simulink model "Farm_FaultBottomBar"  (R2019a)
settings: Solver=ode1  StartTime=0.0  StopTime=1.5  FixedStep=Ts_Power  RelTol=1e-3
PostLoadFcn:
  | %% Init for wind PnO models - global system parameters
  | OVERRIDE_SSN_MEMORY_LIMIT=1;
  | Ts=50e-6;
  | % Ts=50e-10;
  | Ts_Power=Ts;
  | Ts_Control=2*Ts;
  | freq = 50;
  | Fnom=freq;
  | Vac=400e3;
InitFcn:
  | %% Init for wind PnO models - global system parameters
  | OVERRIDE_SSN_MEMORY_LIMIT=1;
  | Ts=50e-6;
  | % Ts=50e-10;
  | Ts_Power=Ts;
  | Ts_Control=2*Ts;
  | freq = 50;
  | Fnom=freq;
  | Vac=400e3;
undefined symbols (not defined in the file or in its folder): D11, Delta, den, DiscIntNeverNeededParam, dx, find_system, gcbh, num, out_Buses, out_WindFarms, sps_rtmsupport
libraries: powerlib x283, simulink x112, powerlib_meascontrol x112, eeSinusoidalMeasurement x76, spsVIMeasurementModel x66, elements x52, simulink_extras x44, eePowerMeasurement x27
(part 17 of 28)

== system Farm_FaultBottomBar/SM_WT1/Wind Type IV Detailed v2.1 - 2/Control/Measurement and Transformation ==
  note: Inputs / filtering
  note: P,Q & V
  note: PLL
  note: Outputs
  note: Check for normal voltage
  note: Protection against unstable grid events
  note: Check for normal frequency
  note: Block forever in case of
      | persistent system overvoltage
  Vabc_grid : Inport
  Iabc_gc : Inport  Port=2
  IL : Inport  Port=3
  Vdc : Inport  Port=4
  Qref : Inport  Port=5
  C_var_filter : Gain  Gain=C_var_filter  SaturateOnIntegerOverflow=on  OutDataTypeStr=Inherit: Same as input  ParamDataTypeStr=Inherit: Same as input
  C_var_filter/Q : Gain  Gain=C_var_filter/Q_filter  SaturateOnIntegerOverflow=on  OutDataTypeStr=Inherit: Same as input  ParamDataTypeStr=Inherit: Same as input
  Compare To Constant1 : simulink/Logic and Bit Operations/Compare To Constant  relop=<  const=0.5  OutDataTypeStr=boolean
  Compare To Constant3 : simulink/Logic and Bit Operations/Compare To Constant  relop=<  const=0.5  OutDataTypeStr=boolean
  Constant : Constant  Value=Vnom
  Constant1 : Constant  Value=Vnom/sqrt(3)*sqrt(2)
  Constant2 : Constant  Value=20
  Constant3 : Constant  SampleTime=Ts
  Constant4 : Constant  SampleTime=Ts
  Digital Clock1 : DigitalClock  SampleTime=Ts
  Digital Clock2 : DigitalClock  SampleTime=Ts
  Discrete 3-phase PLL-Driven Positive-Sequence Active & Reactive Power : Subsystem  mask(Discrete 3-phase PLL-Driven Positive-Sequence Active & Reactive Power){Finit=freq, Fmin=freq*45/60, Par_Vinit=[Vnom/sqrt(3)*sqrt(2) 30], Par_Iinit=[Pnom/sqrt(3)/Vnom*sqrt(2) -10], Ts=Ts}
      mask prompts: Finit "Initial frequency (Hz):"; Fmin "Minimum frequency (Hz):"; Par_Vinit "Voltage initial input: [ Mag  Phase(Degrees) ]"; Par_Iinit "Current initial input: [ Mag  Phase(Degrees) ]"; Ts "Sample time:"
      mask help:
      | This discrete block measures the 3-phase active power P and reactive power Q  associated with a periodic set of 3-phase voltages and currents which may contain harmonics. P and Q are calculated by evaluating the fundamental values (positive-sequence) of the input voltages and currents with a running window over one cycle of the specified frequency (port Freq).
      |  Input port "Sin_Cos" (a two-dimension signal) provides the reference frame required for the computation.
      |
      | input 1: must give the frequency of the fundamental (Hz)
      | Input 2: must contain a  [sin(wt)  cos(wt)] two dimension signal , where w is the rotation speed (rad/s) of the reference frame used for the computation..
      | input 3: Vectorized 3-phase  instantaneous voltage (Vabc)
      | input 4: Vectorized 3-phase instantaneous current (Iabc)
      |
      | Output 1: Vector [Mag_V Mag_I] of the fundamental values (Magnitude) of the voltage & current (peak values of the positive-sequence)
      | Output 2: 3-phase PQ measurement vector [P(W) Q (var)] evaluated at the specified frequency. Current flowing into an RL circuit will produce  positive active and reactive powers.
      |
      | For the first cycle of simulation, the outputs are held constant using the values specified by the parameters "Initial input".
      | he value of the parameter "Minimum frequency" is used to determine the buffer size of the "Variable Transport Delay" block found inside this subsystem.
      mask init:
      | power_initmask();
      settings: OpenFcn=power_openblockproxy();
  Divide : Product  Inputs=*/
  Filter : Subsystem  mask{Freq=Freq_filter, Zeta=Zeta_filter, Ts=Ts}
      mask prompts: Freq "Cut-off frequency (Hz):"; Zeta "Damping factor Zeta:"; Ts "Sample time"
  Gain : Gain  Gain=1.4
  Less Than : RelationalOperator  Operator=>  OutDataTypeStr=boolean  RndMeth=Simplest
  Less Than1 : RelationalOperator  Operator=>  OutDataTypeStr=boolean  RndMeth=Simplest
  Logical Operator : Logic  AllPortsSameDT=off  OutDataTypeStr=boolean
  Math Function1 : Math  Operator=square  SaturateOnIntegerOverflow=on
  Max : MinMax  Inputs=2
  Memory : Memory  InitialCondition=1
  Second-Order Filter1 : powerlib_meascontrol/Filters/Second-Order Filter  FilterType=Lowpass  Fo=50  Zeta=0.707  Ts=Ts  Initialize=off  Vac_Init="[0,  0,  60]"  Vdc_Init=0  PlotResponse=off  FreqRange=[0, 500, 1]
      settings: SourceProductBaseCode=PS
  Selector1 : Selector  InputPortWidth=2  IndexOptions=Index vector (dialog)  Indices=1  OutputSizes=1
  Selector2 : Selector  InputPortWidth=2  IndexOptions=Index vector (dialog)  Indices=1  OutputSizes=1
  Selector3 : Selector  InputPortWidth=2  IndexOptions=Index vector (dialog)  Indices=2  OutputSizes=1
  "Sinusoidal Measurement (PLL, Three-Phase)" : eeSinusoidalMeasurement/Sinusoidal Measurement (PLL, Three-Phase)  Kp_LF=200*0.1  Ki_LF=2000*0.1  F0=freq  Theta0=0  Ts=-1
      settings: SourceProductBaseCode=PS
  Sum : Sum  Inputs=|-+
  Sum1 : Sum  Inputs=|++
  Switch1 : Switch  Criteria=u2 > Threshold
  Switch2 : Switch  Criteria=u2 > Threshold
  Terminator : Terminator
  V->pu : Gain  Gain=1/(Vnom/sqrt(3)*sqrt(2))  SaturateOnIntegerOverflow=on  OutDataTypeStr=Inherit: Same as input  ParamDataTypeStr=Inherit: Same as input
  W->pu : Gain  Gain=-1/Pnom  SaturateOnIntegerOverflow=on  OutDataTypeStr=Inherit: Same as input  ParamDataTypeStr=Inherit: Same as input
  pu->A : Gain  Gain=Pnom/sqrt(3)/Vnom*sqrt(2)  SaturateOnIntegerOverflow=on  OutDataTypeStr=Inherit: Same as input  ParamDataTypeStr=Inherit: Same as input
  pu->V : Gain  Gain=Vnom/sqrt(3)*sqrt(2)  SaturateOnIntegerOverflow=on  OutDataTypeStr=Inherit: Same as input  ParamDataTypeStr=Inherit: Same as input
  "var->pu " : Gain  Gain=-1/Pnom  SaturateOnIntegerOverflow=on  OutDataTypeStr=Inherit: Same as input  ParamDataTypeStr=Inherit: Same as input
  "IL " : Outport  VectorParamsAs1DForOutWhenUnconnected=on
  Theta_PLL : Outport  Port=2  VectorParamsAs1DForOutWhenUnconnected=on
  Pmeas : Outport  Port=3  VectorParamsAs1DForOutWhenUnconnected=on
  Qmeas : Outport  Port=4  VectorParamsAs1DForOutWhenUnconnected=on
  Vmag : Outport  Port=5  VectorParamsAs1DForOutWhenUnconnected=on
  Vdc_meas : Outport  Port=6  VectorParamsAs1DForOutWhenUnconnected=on
  Qref_pu : Outport  Port=7  VectorParamsAs1DForOutWhenUnconnected=on
  Vnormal : Outport  Port=8  VectorParamsAs1DForOutWhenUnconnected=on
  wires:
  [IL] -> "IL "/1
  Filter/3("IL ") -> [IL]
  IL/1 -> Filter/3(IL)
  Sum1/1 -> W->pu/1
  C_var_filter/Q/1 -> Sum1/2
  Selector1/1 -> Sum1/1
  Math Function1/1 -> C_var_filter/1, C_var_filter/Q/1
  Sum/1 -> "var->pu "/1  "Q meas"
  C_var_filter/1 -> Sum/1
  Selector3/1 -> Sum/2  "Q grid"
  Divide/1 -> Math Function1/1
  Constant1/1 -> Divide/2
  [V_volt] -> Divide/1
  Iabc_gc/1 -> Filter/2(Iabc_grid_conv)
  Filter/5("Qref ") -> [Qref]
  Filter/4("Vdc ") -> [Vdc_meas]
  Filter/2("Iabc_grid_conv ") -> [Iabc_gc]
  Filter/1("Vabc_grid ") -> [Vabc_grid]
  Qref/1 -> Filter/5(Qref)
  Vdc/1 -> Filter/4(Vdc)
  Vabc_grid/1 -> Filter/1(Vabc_grid)
  Discrete 3-phase PLL-Driven Positive-Sequence Active & Reactive Power/2(P_Q) -> [PQ]
  [Iabc_gc] -> pu->A/1
  [Qref] -> Qref_pu/1
  [Vdc_meas] -> Vdc_meas/1
  [PQ] -> Selector1/1
  pu->A/1 -> Discrete 3-phase PLL-Driven Positive-Sequence Active & Reactive Power/4(Iabc)
  [Vmeas] -> Vmag/1
  [Pmeas] -> Pmeas/1
  [Theta] -> Theta_PLL/1
  [Vabc_grid] -> "Sinusoidal Measurement (PLL, Three-Phase)"/1
  [Theta] -> Discrete 3-phase PLL-Driven Positive-Sequence Active & Reactive Power/2(w)
  "Sinusoidal Measurement (PLL, Three-Phase)"/2 -> [Theta]
  W->pu/1 -> [Pmeas]
  pu->V/1 -> Discrete 3-phase PLL-Driven Positive-Sequence Active & Reactive Power/3(Vabc)
  "Sinusoidal Measurement (PLL, Three-Phase)"/1 -> [Freq]
  Discrete 3-phase PLL-Driven Positive-Sequence Active & Reactive Power/1(Mag_V_I) -> Selector2/1
  [V_volt] -> V->pu/1
  V->pu/1 -> [Vmeas]
  [PQ] -> Selector3/1
  "var->pu "/1 -> [Qmeas]  "Q meas pu"
  [Qmeas] -> Qmeas/1
  "Sinusoidal Measurement (PLL, Three-Phase)"/3 -> Terminator/1
  Selector2/1 -> [V_volt]  "V volt"
  [Vabc_grid] -> pu->V/1
  [Vnormal] -> Vnormal/1
  [Freq] -> Discrete 3-phase PLL-Driven Positive-Sequence Active & Reactive Power/1(Freq)
  [V_volt] -> Second-Order Filter1/1
  Constant2/1 -> Less Than1/2  "20 Hz"
  [Freq] -> Less Than1/1  "Freq"
  Memory/1 -> Max/2
  Gain/1 -> Less Than/1
  Second-Order Filter1/1 -> Less Than/2
  Constant/1 -> Gain/1
  Max/1 -> [Vnormal], Memory/1
  Logical Operator/1 -> Max/1
  Constant3/1 -> Switch2/1
  Digital Clock1/1 -> Compare To Constant3/1
  Compare To Constant3/1 -> Switch2/2
  Less Than/1 -> Switch2/3
  Switch2/1 -> Logical Operator/1  "test1"
  Digital Clock2/1 -> Compare To Constant1/1
  Constant4/1 -> Switch1/1
  Less Than1/1 -> Switch1/3  "Comparator freq"
  Switch1/1 -> Logical Operator/2  "test2"
  Compare To Constant1/1 -> Switch1/2

== system Farm_FaultBottomBar/SM_WT1/Wind Type IV Detailed v2.1 - 2/Control/PI_P ==
  u : Inport
  Enable : EnablePort
  Discrete PID Controller2 : simulink/Continuous/PID Controller  Controller=PI  Form=Parallel  TimeDomain=Discrete-time  SampleTime=-1  IntegratorMethod=Forward Euler  FilterMethod=Forward Euler  ControllerParametersSource=internal  P=5  I=30  D=2  UseFilter=on  N=100  TunerSelectOption=Transfer Function Based (PID Tuner App)  InitialConditionSource=internal  InitialConditionForIntegrator=0  InitialConditionForFilter=0  DifferentiatorICPrevScaledInput=0  ExternalReset=none  TrackingMode=off  Kt=1  LimitOutput=on  UpperSaturationLimit=0.8  LowerSaturationLimit=-0.8  LinearizeAsGain=off  AntiWindupMode=none  Kb=1  POutMin=[]  POutMax=[]  IOutMin=[]  IOutMax=[]  DOutMin=[]  DOutMax=[]  NOutMin=[]  NOutMax=[]  SumOutMin=[]  SumOutMax=[]  SaturationOutMin=[]  SaturationOutMax=[]  PParamMin=[]  PParamMax=[]  IParamMin=[]  IParamMax=[]  DParamMin=[]  DParamMax=[]  NParamMin=[]  NParamMax=[]  KbParamMin=[]  KbParamMax=[]  KtParamMin=[]  KtParamMax=[]  KbOutMin=[]  KbOutMax=[]  KtOutMin=[]  KtOutMax=[]  IntegratorOutMin=[]  IntegratorOutMax=[]  FilterOutMin=[]  FilterOutMax=[]  SumI1OutMin=[]  SumI1OutMax=[]  SumI2OutMin=[]  SumI2OutMax=[]  SumI3OutMin=[]  SumI3OutMax=[]  SumI4OutMin=[]  SumI4OutMax=[]  SumDOutMin=[]  SumDOutMax=[]  DifferentiatorOutMin=[]  DifferentiatorOutMax=[]  FilterDiffOutCoefMin=[]  FilterDiffOutCoefMax=[]  ReciprocalOutMin=[]  ReciprocalOutMax=[]  SumDenOutMin=[]  SumDenOutMax=[]  SumNumOutMin=[]  SumNumOutMax=[]  DivideOutMin=[]  DivideOutMax=[]  IntegratorContinuousStateAttributes=''  IntegratorStateMustResolveToSignalObject=off  IntegratorRTWStateStorageClass=Auto  FilterContinuousStateAttributes=''  FilterStateMustResolveToSignalObject=off  FilterRTWStateStorageClass=Auto  ParallelPVariant=InternalParameters  IdealPVariant=Disabled  IVariant=InternalParameters  DVariant=Disabled  IntegratorVariant=Discrete  SatVariant=Enabled  AWVariant=Passthrough  PCopyVariant=Disabled  TRVariant=Disabled  FdbkBlocksVariant=Forward  IdealPFdbkVariant=Disabled  SatFdbkVariant=Disabled  DerivativeFilterVariant=Disabled  NVariant=Disabled  NCopyVariant=Disabled_SignalSpec  FilterICVariant=Disabled  IntegratorICVariant=InternalICs  ExternalResetVariant=Disabled  TRSumVariant=Passthrough  SumFdbkVariant=Disabled  SumVariant=Sum_PI
  PI_out : Outport  VectorParamsAs1DForOutWhenUnconnected=on
  wires:
  Discrete PID Controller2/1 -> PI_out/1  "d PI_out"
  u/1 -> Discrete PID Controller2/1

== system Farm_FaultBottomBar/SM_WT1/Wind Type IV Detailed v2.1 - 2/Control/PI_Q ==
  Qerr : Inport
  Enable : EnablePort
  Discrete PID Controller1 : simulink/Continuous/PID Controller  Controller=PI  Form=Parallel  TimeDomain=Discrete-time  SampleTime=-1  IntegratorMethod=Forward Euler  FilterMethod=Forward Euler  ControllerParametersSource=internal  P=0.5  I=8  D=2  UseFilter=on  N=100  TunerSelectOption=Transfer Function Based (PID Tuner App)  InitialConditionSource=internal  InitialConditionForIntegrator=0  InitialConditionForFilter=0  DifferentiatorICPrevScaledInput=0  ExternalReset=none  TrackingMode=off  Kt=1  LimitOutput=off  UpperSaturationLimit=inf  LowerSaturationLimit=-inf  LinearizeAsGain=off  AntiWindupMode=none  Kb=1  POutMin=[]  POutMax=[]  IOutMin=[]  IOutMax=[]  DOutMin=[]  DOutMax=[]  NOutMin=[]  NOutMax=[]  SumOutMin=[]  SumOutMax=[]  SaturationOutMin=[]  SaturationOutMax=[]  PParamMin=[]  PParamMax=[]  IParamMin=[]  IParamMax=[]  DParamMin=[]  DParamMax=[]  NParamMin=[]  NParamMax=[]  KbParamMin=[]  KbParamMax=[]  KtParamMin=[]  KtParamMax=[]  KbOutMin=[]  KbOutMax=[]  KtOutMin=[]  KtOutMax=[]  IntegratorOutMin=[]  IntegratorOutMax=[]  FilterOutMin=[]  FilterOutMax=[]  SumI1OutMin=[]  SumI1OutMax=[]  SumI2OutMin=[]  SumI2OutMax=[]  SumI3OutMin=[]  SumI3OutMax=[]  SumI4OutMin=[]  SumI4OutMax=[]  SumDOutMin=[]  SumDOutMax=[]  DifferentiatorOutMin=[]  DifferentiatorOutMax=[]  FilterDiffOutCoefMin=[]  FilterDiffOutCoefMax=[]  ReciprocalOutMin=[]  ReciprocalOutMax=[]  SumDenOutMin=[]  SumDenOutMax=[]  SumNumOutMin=[]  SumNumOutMax=[]  DivideOutMin=[]  DivideOutMax=[]  IntegratorContinuousStateAttributes=''  IntegratorStateMustResolveToSignalObject=off  IntegratorRTWStateStorageClass=Auto  FilterContinuousStateAttributes=''  FilterStateMustResolveToSignalObject=off  FilterRTWStateStorageClass=Auto  ParallelPVariant=InternalParameters  IdealPVariant=Disabled  IVariant=InternalParameters  DVariant=Disabled  IntegratorVariant=Discrete  SatVariant=Disabled  AWVariant=Passthrough  PCopyVariant=Disabled  TRVariant=Disabled  FdbkBlocksVariant=Forward  IdealPFdbkVariant=Disabled  SatFdbkVariant=Disabled  DerivativeFilterVariant=Disabled  NVariant=Disabled  NCopyVariant=Disabled_SignalSpec  FilterICVariant=Disabled  IntegratorICVariant=InternalICs  ExternalResetVariant=Disabled  TRSumVariant=Passthrough  SumFdbkVariant=Disabled  SumVariant=Sum_PI
  PI_out : Outport  VectorParamsAs1DForOutWhenUnconnected=on
  wires:
  Discrete PID Controller1/1 -> PI_out/1  "q PI_out"
  Qerr/1 -> Discrete PID Controller1/1

== system Farm_FaultBottomBar/SM_WT1/Wind Type IV Detailed v2.1 - 2/Control/Pulse Generator1 ==
  Duty_Cycle : Inport
  Add : Sum  Inputs=-+
  Constant3 : Constant
  Constant4 : Constant  Value=0
  Digital Clock : DigitalClock  SampleTime=Ts
  Divide2 : Product  Inputs=**
  Divide3 : Product  Inputs=**
  Math Function : Math  Operator=mod  SaturateOnIntegerOverflow=on
  Nb_of_samples_by_cycle : Constant  Value=1/Freq_sawtooth/Ts
  Relational Operator1 : RelationalOperator  Operator=>  OutDataTypeStr=boolean  RndMeth=Nearest
  Rounding Function1 : Rounding  Operator=round
  Switch : Switch  Threshold=0.5
  Ts : Constant  Value=Ts
  Pulse : Outport  VectorParamsAs1DForOutWhenUnconnected=on
  wires:
  Switch/1 -> Pulse/1
  Add/1 -> Divide2/2
  Digital Clock/1 -> Math Function/1
  Ts/1 -> Add/1, Divide3/1
  Rounding Function1/1 -> Divide3/2  "Nb_of_samples_by_cycle"
  Duty_Cycle/1 -> Divide2/1
  Divide3/1 -> Math Function/2, Add/2  "Period_of_cycle"
  Divide2/1 -> Relational Operator1/1
  Nb_of_samples_by_cycle/1 -> Rounding Function1/1
  Relational Operator1/1 -> Switch/2
  Constant3/1 -> Switch/1
  Constant4/1 -> Switch/3
  Math Function/1 -> Relational Operator1/2

== system Farm_FaultBottomBar/SM_WT1/Wind Type IV Detailed v2.1 - 24/AC fault ride though characteristic/Triggered Subsystem ==
  In1 : Inport
  Trigger : TriggerPort  VariantControl=Variant
  Time_trigger_FRT : Outport  VectorParamsAs1DForOutWhenUnconnected=on
  wires:
  In1/1 -> Time_trigger_FRT/1

== system Farm_FaultBottomBar/SM_WT1/Wind Type IV Detailed v2.1 - 24/Control/2 sample av. ==
  in : Inport
  Delay : Delay  DelayLength=1  InitialCondition=Init_value  SampleTime=Ts
  Delay1 : Delay  DelayLength=1  InitialCondition=Init_value  SampleTime=Ts
  Gain : Gain  Gain=0.5
  Sum1 : Sum  Inputs=|++
  out : Outport
  wires:
  Gain/1 -> out/1
  in/1 -> Delay/1
  Delay1/1 -> Sum1/2
  Sum1/1 -> Gain/1
  Delay/1 -> Delay1/1, Sum1/1

== system Farm_FaultBottomBar/SM_WT1/Wind Type IV Detailed v2.1 - 24/Control/Measurement and Transformation ==
  note: Block forever in case of
      | persistent system overvoltage
  note: Check for normal frequency
  note: Protection against unstable grid events
  note: Check for normal voltage
  note: Outputs
  note: PLL
  note: P,Q & V
  note: Inputs / filtering
  Vabc_grid : Inport
  Iabc_gc : Inport  Port=2
  IL : Inport  Port=3
  Vdc : Inport  Port=4
  Qref : Inport  Port=5
  C_var_filter : Gain  Gain=C_var_filter  SaturateOnIntegerOverflow=on  OutDataTypeStr=Inherit: Same as input  ParamDataTypeStr=Inherit: Same as input
  C_var_filter/Q : Gain  Gain=C_var_filter/Q_filter  SaturateOnIntegerOverflow=on  OutDataTypeStr=Inherit: Same as input  ParamDataTypeStr=Inherit: Same as input
  Compare To Constant1 : simulink/Logic and Bit Operations/Compare To Constant  relop=<  const=0.5  OutDataTypeStr=boolean
  Compare To Constant3 : simulink/Logic and Bit Operations/Compare To Constant  relop=<  const=0.5  OutDataTypeStr=boolean
  Constant : Constant  Value=Vnom
  Constant1 : Constant  Value=Vnom/sqrt(3)*sqrt(2)
  Constant2 : Constant  Value=20
  Constant3 : Constant  SampleTime=Ts
  Constant4 : Constant  SampleTime=Ts
  Digital Clock1 : DigitalClock  SampleTime=Ts
  Digital Clock2 : DigitalClock  SampleTime=Ts
  Discrete 3-phase PLL-Driven Positive-Sequence Active & Reactive Power : Subsystem  mask(Discrete 3-phase PLL-Driven Positive-Sequence Active & Reactive Power){Finit=freq, Fmin=freq*45/60, Par_Vinit=[Vnom/sqrt(3)*sqrt(2) 30], Par_Iinit=[Pnom/sqrt(3)/Vnom*sqrt(2) -10], Ts=Ts}
      mask prompts: Finit "Initial frequency (Hz):"; Fmin "Minimum frequency (Hz):"; Par_Vinit "Voltage initial input: [ Mag  Phase(Degrees) ]"; Par_Iinit "Current initial input: [ Mag  Phase(Degrees) ]"; Ts "Sample time:"
      mask help:
      | This discrete block measures the 3-phase active power P and reactive power Q  associated with a periodic set of 3-phase voltages and currents which may contain harmonics. P and Q are calculated by evaluating the fundamental values (positive-sequence) of the input voltages and currents with a running window over one cycle of the specified frequency (port Freq).
      |  Input port "Sin_Cos" (a two-dimension signal) provides the reference frame required for the computation.
      |
      | input 1: must give the frequency of the fundamental (Hz)
      | Input 2: must contain a  [sin(wt)  cos(wt)] two dimension signal , where w is the rotation speed (rad/s) of the reference frame used for the computation..
      | input 3: Vectorized 3-phase  instantaneous voltage (Vabc)
      | input 4: Vectorized 3-phase instantaneous current (Iabc)
      |
      | Output 1: Vector [Mag_V Mag_I] of the fundamental values (Magnitude) of the voltage & current (peak values of the positive-sequence)
      | Output 2: 3-phase PQ measurement vector [P(W) Q (var)] evaluated at the specified frequency. Current flowing into an RL circuit will produce  positive active and reactive powers.
      |
      | For the first cycle of simulation, the outputs are held constant using the values specified by the parameters "Initial input".
      | he value of the parameter "Minimum frequency" is used to determine the buffer size of the "Variable Transport Delay" block found inside this subsystem.
      mask init:
      | power_initmask();
      settings: OpenFcn=power_openblockproxy();
  Divide : Product  Inputs=*/
  Filter : Subsystem  mask{Freq=Freq_filter, Zeta=Zeta_filter, Ts=Ts}
      mask prompts: Freq "Cut-off frequency (Hz):"; Zeta "Damping factor Zeta:"; Ts "Sample time"
  Gain : Gain  Gain=1.4
  Less Than : RelationalOperator  Operator=>  OutDataTypeStr=boolean  RndMeth=Simplest
  Less Than1 : RelationalOperator  Operator=>  OutDataTypeStr=boolean  RndMeth=Simplest
  Logical Operator : Logic  AllPortsSameDT=off  OutDataTypeStr=boolean
  Math Function1 : Math  Operator=square  SaturateOnIntegerOverflow=on
  Max : MinMax  Inputs=2
  Memory : Memory  InitialCondition=1
  Second-Order Filter1 : powerlib_meascontrol/Filters/Second-Order Filter  FilterType=Lowpass  Fo=50  Zeta=0.707  Ts=Ts  Initialize=off  Vac_Init="[0,  0,  60]"  Vdc_Init=0  PlotResponse=off  FreqRange=[0, 500, 1]
      settings: SourceProductBaseCode=PS
  Selector1 : Selector  InputPortWidth=2  IndexOptions=Index vector (dialog)  Indices=1  OutputSizes=1
  Selector2 : Selector  InputPortWidth=2  IndexOptions=Index vector (dialog)  Indices=1  OutputSizes=1
  Selector3 : Selector  InputPortWidth=2  IndexOptions=Index vector (dialog)  Indices=2  OutputSizes=1
  "Sinusoidal Measurement (PLL, Three-Phase)" : eeSinusoidalMeasurement/Sinusoidal Measurement (PLL, Three-Phase)  Kp_LF=200*0.1  Ki_LF=2000*0.1  F0=freq  Theta0=0  Ts=-1
      settings: SourceProductBaseCode=PS
  Sum : Sum  Inputs=|-+
  Sum1 : Sum  Inputs=|++
  Switch1 : Switch  Criteria=u2 > Threshold
  Switch2 : Switch  Criteria=u2 > Threshold
  Terminator : Terminator
  V->pu : Gain  Gain=1/(Vnom/sqrt(3)*sqrt(2))  SaturateOnIntegerOverflow=on  OutDataTypeStr=Inherit: Same as input  ParamDataTypeStr=Inherit: Same as input
  W->pu : Gain  Gain=-1/Pnom  SaturateOnIntegerOverflow=on  OutDataTypeStr=Inherit: Same as input  ParamDataTypeStr=Inherit: Same as input
  pu->A : Gain  Gain=Pnom/sqrt(3)/Vnom*sqrt(2)  SaturateOnIntegerOverflow=on  OutDataTypeStr=Inherit: Same as input  ParamDataTypeStr=Inherit: Same as input
  pu->V : Gain  Gain=Vnom/sqrt(3)*sqrt(2)  SaturateOnIntegerOverflow=on  OutDataTypeStr=Inherit: Same as input  ParamDataTypeStr=Inherit: Same as input
  "var->pu " : Gain  Gain=-1/Pnom  SaturateOnIntegerOverflow=on  OutDataTypeStr=Inherit: Same as input  ParamDataTypeStr=Inherit: Same as input
  "IL " : Outport  VectorParamsAs1DForOutWhenUnconnected=on
  Theta_PLL : Outport  Port=2  VectorParamsAs1DForOutWhenUnconnected=on
  Pmeas : Outport  Port=3  VectorParamsAs1DForOutWhenUnconnected=on
  Qmeas : Outport  Port=4  VectorParamsAs1DForOutWhenUnconnected=on
  Vmag : Outport  Port=5  VectorParamsAs1DForOutWhenUnconnected=on
  Vdc_meas : Outport  Port=6  VectorParamsAs1DForOutWhenUnconnected=on
  Qref_pu : Outport  Port=7  VectorParamsAs1DForOutWhenUnconnected=on
  Vnormal : Outport  Port=8  VectorParamsAs1DForOutWhenUnconnected=on
  wires:
  Compare To Constant1/1 -> Switch1/2
  Switch1/1 -> Logical Operator/2  "test2"
  Less Than1/1 -> Switch1/3  "Comparator freq"
  Constant4/1 -> Switch1/1
  Digital Clock2/1 -> Compare To Constant1/1
  Switch2/1 -> Logical Operator/1  "test1"
  Less Than/1 -> Switch2/3
  Compare To Constant3/1 -> Switch2/2
  Digital Clock1/1 -> Compare To Constant3/1
  Constant3/1 -> Switch2/1
  Logical Operator/1 -> Max/1
  Max/1 -> Memory/1, [Vnormal]
  Constant/1 -> Gain/1
  Second-Order Filter1/1 -> Less Than/2
  Gain/1 -> Less Than/1
  Memory/1 -> Max/2
  [Freq] -> Less Than1/1  "Freq"
  Constant2/1 -> Less Than1/2  "20 Hz"
  [V_volt] -> Second-Order Filter1/1
  [Freq] -> Discrete 3-phase PLL-Driven Positive-Sequence Active & Reactive Power/1(Freq)
  [Vnormal] -> Vnormal/1
  [Vabc_grid] -> pu->V/1
  Selector2/1 -> [V_volt]  "V volt"
  "Sinusoidal Measurement (PLL, Three-Phase)"/3 -> Terminator/1
  [Qmeas] -> Qmeas/1
  "var->pu "/1 -> [Qmeas]  "Q meas pu"
  [PQ] -> Selector3/1
  V->pu/1 -> [Vmeas]
  [V_volt] -> V->pu/1
  Discrete 3-phase PLL-Driven Positive-Sequence Active & Reactive Power/1(Mag_V_I) -> Selector2/1
  "Sinusoidal Measurement (PLL, Three-Phase)"/1 -> [Freq]
  pu->V/1 -> Discrete 3-phase PLL-Driven Positive-Sequence Active & Reactive Power/3(Vabc)
  W->pu/1 -> [Pmeas]
  "Sinusoidal Measurement (PLL, Three-Phase)"/2 -> [Theta]
  [Theta] -> Discrete 3-phase PLL-Driven Positive-Sequence Active & Reactive Power/2(w)
  [Vabc_grid] -> "Sinusoidal Measurement (PLL, Three-Phase)"/1
  [Theta] -> Theta_PLL/1
  [Pmeas] -> Pmeas/1
  [Vmeas] -> Vmag/1
  pu->A/1 -> Discrete 3-phase PLL-Driven Positive-Sequence Active & Reactive Power/4(Iabc)
  [PQ] -> Selector1/1
  [Vdc_meas] -> Vdc_meas/1
  [Qref] -> Qref_pu/1
  [Iabc_gc] -> pu->A/1
  Discrete 3-phase PLL-Driven Positive-Sequence Active & Reactive Power/2(P_Q) -> [PQ]
  Vabc_grid/1 -> Filter/1(Vabc_grid)
  Vdc/1 -> Filter/4(Vdc)
  Qref/1 -> Filter/5(Qref)
  Filter/1("Vabc_grid ") -> [Vabc_grid]
  Filter/2("Iabc_grid_conv ") -> [Iabc_gc]
  Filter/4("Vdc ") -> [Vdc_meas]
  Filter/5("Qref ") -> [Qref]
  Iabc_gc/1 -> Filter/2(Iabc_grid_conv)
  [V_volt] -> Divide/1
  Constant1/1 -> Divide/2
  Divide/1 -> Math Function1/1
  Selector3/1 -> Sum/2  "Q grid"
  C_var_filter/1 -> Sum/1
  Sum/1 -> "var->pu "/1  "Q meas"
  Math Function1/1 -> C_var_filter/Q/1, C_var_filter/1
  Selector1/1 -> Sum1/1
  C_var_filter/Q/1 -> Sum1/2
  Sum1/1 -> W->pu/1
  IL/1 -> Filter/3(IL)
  Filter/3("IL ") -> [IL]
  [IL] -> "IL "/1

== system Farm_FaultBottomBar/SM_WT1/Wind Type IV Detailed v2.1 - 24/Control/PI_P ==
  u : Inport
  Enable : EnablePort
  Discrete PID Controller2 : simulink/Continuous/PID Controller  Controller=PI  Form=Parallel  TimeDomain=Discrete-time  SampleTime=-1  IntegratorMethod=Forward Euler  FilterMethod=Forward Euler  ControllerParametersSource=internal  P=5  I=30  D=2  UseFilter=on  N=100  TunerSelectOption=Transfer Function Based (PID Tuner App)  InitialConditionSource=internal  InitialConditionForIntegrator=0  InitialConditionForFilter=0  DifferentiatorICPrevScaledInput=0  ExternalReset=none  TrackingMode=off  Kt=1  LimitOutput=on  UpperSaturationLimit=0.8  LowerSaturationLimit=-0.8  LinearizeAsGain=off  AntiWindupMode=none  Kb=1  POutMin=[]  POutMax=[]  IOutMin=[]  IOutMax=[]  DOutMin=[]  DOutMax=[]  NOutMin=[]  NOutMax=[]  SumOutMin=[]  SumOutMax=[]  SaturationOutMin=[]  SaturationOutMax=[]  PParamMin=[]  PParamMax=[]  IParamMin=[]  IParamMax=[]  DParamMin=[]  DParamMax=[]  NParamMin=[]  NParamMax=[]  KbParamMin=[]  KbParamMax=[]  KtParamMin=[]  KtParamMax=[]  KbOutMin=[]  KbOutMax=[]  KtOutMin=[]  KtOutMax=[]  IntegratorOutMin=[]  IntegratorOutMax=[]  FilterOutMin=[]  FilterOutMax=[]  SumI1OutMin=[]  SumI1OutMax=[]  SumI2OutMin=[]  SumI2OutMax=[]  SumI3OutMin=[]  SumI3OutMax=[]  SumI4OutMin=[]  SumI4OutMax=[]  SumDOutMin=[]  SumDOutMax=[]  DifferentiatorOutMin=[]  DifferentiatorOutMax=[]  FilterDiffOutCoefMin=[]  FilterDiffOutCoefMax=[]  ReciprocalOutMin=[]  ReciprocalOutMax=[]  SumDenOutMin=[]  SumDenOutMax=[]  SumNumOutMin=[]  SumNumOutMax=[]  DivideOutMin=[]  DivideOutMax=[]  IntegratorContinuousStateAttributes=''  IntegratorStateMustResolveToSignalObject=off  IntegratorRTWStateStorageClass=Auto  FilterContinuousStateAttributes=''  FilterStateMustResolveToSignalObject=off  FilterRTWStateStorageClass=Auto  ParallelPVariant=InternalParameters  IdealPVariant=Disabled  IVariant=InternalParameters  DVariant=Disabled  IntegratorVariant=Discrete  SatVariant=Enabled  AWVariant=Passthrough  PCopyVariant=Disabled  TRVariant=Disabled  FdbkBlocksVariant=Forward  IdealPFdbkVariant=Disabled  SatFdbkVariant=Disabled  DerivativeFilterVariant=Disabled  NVariant=Disabled  NCopyVariant=Disabled_SignalSpec  FilterICVariant=Disabled  IntegratorICVariant=InternalICs  ExternalResetVariant=Disabled  TRSumVariant=Passthrough  SumFdbkVariant=Disabled  SumVariant=Sum_PI
  PI_out : Outport  VectorParamsAs1DForOutWhenUnconnected=on
  wires:
  u/1 -> Discrete PID Controller2/1
  Discrete PID Controller2/1 -> PI_out/1  "d PI_out"

== system Farm_FaultBottomBar/SM_WT1/Wind Type IV Detailed v2.1 - 24/Control/PI_Q ==
  Qerr : Inport
  Enable : EnablePort
  Discrete PID Controller1 : simulink/Continuous/PID Controller  Controller=PI  Form=Parallel  TimeDomain=Discrete-time  SampleTime=-1  IntegratorMethod=Forward Euler  FilterMethod=Forward Euler  ControllerParametersSource=internal  P=0.5  I=8  D=2  UseFilter=on  N=100  TunerSelectOption=Transfer Function Based (PID Tuner App)  InitialConditionSource=internal  InitialConditionForIntegrator=0  InitialConditionForFilter=0  DifferentiatorICPrevScaledInput=0  ExternalReset=none  TrackingMode=off  Kt=1  LimitOutput=off  UpperSaturationLimit=inf  LowerSaturationLimit=-inf  LinearizeAsGain=off  AntiWindupMode=none  Kb=1  POutMin=[]  POutMax=[]  IOutMin=[]  IOutMax=[]  DOutMin=[]  DOutMax=[]  NOutMin=[]  NOutMax=[]  SumOutMin=[]  SumOutMax=[]  SaturationOutMin=[]  SaturationOutMax=[]  PParamMin=[]  PParamMax=[]  IParamMin=[]  IParamMax=[]  DParamMin=[]  DParamMax=[]  NParamMin=[]  NParamMax=[]  KbParamMin=[]  KbParamMax=[]  KtParamMin=[]  KtParamMax=[]  KbOutMin=[]  KbOutMax=[]  KtOutMin=[]  KtOutMax=[]  IntegratorOutMin=[]  IntegratorOutMax=[]  FilterOutMin=[]  FilterOutMax=[]  SumI1OutMin=[]  SumI1OutMax=[]  SumI2OutMin=[]  SumI2OutMax=[]  SumI3OutMin=[]  SumI3OutMax=[]  SumI4OutMin=[]  SumI4OutMax=[]  SumDOutMin=[]  SumDOutMax=[]  DifferentiatorOutMin=[]  DifferentiatorOutMax=[]  FilterDiffOutCoefMin=[]  FilterDiffOutCoefMax=[]  ReciprocalOutMin=[]  ReciprocalOutMax=[]  SumDenOutMin=[]  SumDenOutMax=[]  SumNumOutMin=[]  SumNumOutMax=[]  DivideOutMin=[]  DivideOutMax=[]  IntegratorContinuousStateAttributes=''  IntegratorStateMustResolveToSignalObject=off  IntegratorRTWStateStorageClass=Auto  FilterContinuousStateAttributes=''  FilterStateMustResolveToSignalObject=off  FilterRTWStateStorageClass=Auto  ParallelPVariant=InternalParameters  IdealPVariant=Disabled  IVariant=InternalParameters  DVariant=Disabled  IntegratorVariant=Discrete  SatVariant=Disabled  AWVariant=Passthrough  PCopyVariant=Disabled  TRVariant=Disabled  FdbkBlocksVariant=Forward  IdealPFdbkVariant=Disabled  SatFdbkVariant=Disabled  DerivativeFilterVariant=Disabled  NVariant=Disabled  NCopyVariant=Disabled_SignalSpec  FilterICVariant=Disabled  IntegratorICVariant=InternalICs  ExternalResetVariant=Disabled  TRSumVariant=Passthrough  SumFdbkVariant=Disabled  SumVariant=Sum_PI
  PI_out : Outport  VectorParamsAs1DForOutWhenUnconnected=on
  wires:
  Qerr/1 -> Discrete PID Controller1/1
  Discrete PID Controller1/1 -> PI_out/1  "q PI_out"

== system Farm_FaultBottomBar/SM_WT1/Wind Type IV Detailed v2.1 - 24/Control/Pulse Generator1 ==
  Duty_Cycle : Inport
  Add : Sum  Inputs=-+
  Constant3 : Constant
  Constant4 : Constant  Value=0
  Digital Clock : DigitalClock  SampleTime=Ts
  Divide2 : Product  Inputs=**
  Divide3 : Product  Inputs=**
  Math Function : Math  Operator=mod  SaturateOnIntegerOverflow=on
  Nb_of_samples_by_cycle : Constant  Value=1/Freq_sawtooth/Ts
  Relational Operator1 : RelationalOperator  Operator=>  OutDataTypeStr=boolean  RndMeth=Nearest
  Rounding Function1 : Rounding  Operator=round
  Switch : Switch  Threshold=0.5
  Ts : Constant  Value=Ts
  Pulse : Outport  VectorParamsAs1DForOutWhenUnconnected=on
  wires:
  Math Function/1 -> Relational Operator1/2
  Constant4/1 -> Switch/3
  Constant3/1 -> Switch/1
  Relational Operator1/1 -> Switch/2
  Nb_of_samples_by_cycle/1 -> Rounding Function1/1
  Divide2/1 -> Relational Operator1/1
  Divide3/1 -> Add/2, Math Function/2  "Period_of_cycle"
  Duty_Cycle/1 -> Divide2/1
  Rounding Function1/1 -> Divide3/2  "Nb_of_samples_by_cycle"
  Ts/1 -> Divide3/1, Add/1
  Digital Clock/1 -> Math Function/1
  Add/1 -> Divide2/2
  Switch/1 -> Pulse/1

== system Farm_FaultBottomBar/SM_WT1/Wind Type IV Detailed v2.1 - 3/AC fault ride though characteristic/Triggered Subsystem ==
  In1 : Inport
  Trigger : TriggerPort  VariantControl=Variant
  Time_trigger_FRT : Outport  VectorParamsAs1DForOutWhenUnconnected=on
  wires:
  In1/1 -> Time_trigger_FRT/1

== system Farm_FaultBottomBar/SM_WT1/Wind Type IV Detailed v2.1 - 3/Control/2 sample av. ==
  in : Inport
  Delay : Delay  DelayLength=1  InitialCondition=Init_value  SampleTime=Ts
  Delay1 : Delay  DelayLength=1  InitialCondition=Init_value  SampleTime=Ts
  Gain : Gain  Gain=0.5
  Sum1 : Sum  Inputs=|++
  out : Outport
  wires:
  Delay/1 -> Sum1/1, Delay1/1
  Sum1/1 -> Gain/1
  Delay1/1 -> Sum1/2
  in/1 -> Delay/1
  Gain/1 -> out/1

== system Farm_FaultBottomBar/SM_WT1/Wind Type IV Detailed v2.1 - 3/Control/Measurement and Transformation ==
  note: Inputs / filtering
  note: P,Q & V
  note: PLL
  note: Outputs
  note: Check for normal voltage
  note: Protection against unstable grid events
  note: Check for normal frequency
  note: Block forever in case of
      | persistent system overvoltage
  Vabc_grid : Inport
  Iabc_gc : Inport  Port=2
  IL : Inport  Port=3
  Vdc : Inport  Port=4
  Qref : Inport  Port=5
  C_var_filter : Gain  Gain=C_var_filter  SaturateOnIntegerOverflow=on  OutDataTypeStr=Inherit: Same as input  ParamDataTypeStr=Inherit: Same as input
  C_var_filter/Q : Gain  Gain=C_var_filter/Q_filter  SaturateOnIntegerOverflow=on  OutDataTypeStr=Inherit: Same as input  ParamDataTypeStr=Inherit: Same as input
  Compare To Constant1 : simulink/Logic and Bit Operations/Compare To Constant  relop=<  const=0.5  OutDataTypeStr=boolean
  Compare To Constant3 : simulink/Logic and Bit Operations/Compare To Constant  relop=<  const=0.5  OutDataTypeStr=boolean
  Constant : Constant  Value=Vnom
  Constant1 : Constant  Value=Vnom/sqrt(3)*sqrt(2)
  Constant2 : Constant  Value=20
  Constant3 : Constant  SampleTime=Ts
  Constant4 : Constant  SampleTime=Ts
  Digital Clock1 : DigitalClock  SampleTime=Ts
  Digital Clock2 : DigitalClock  SampleTime=Ts
  Discrete 3-phase PLL-Driven Positive-Sequence Active & Reactive Power : Subsystem  mask(Discrete 3-phase PLL-Driven Positive-Sequence Active & Reactive Power){Finit=freq, Fmin=freq*45/60, Par_Vinit=[Vnom/sqrt(3)*sqrt(2) 30], Par_Iinit=[Pnom/sqrt(3)/Vnom*sqrt(2) -10], Ts=Ts}
      mask prompts: Finit "Initial frequency (Hz):"; Fmin "Minimum frequency (Hz):"; Par_Vinit "Voltage initial input: [ Mag  Phase(Degrees) ]"; Par_Iinit "Current initial input: [ Mag  Phase(Degrees) ]"; Ts "Sample time:"
      mask help:
      | This discrete block measures the 3-phase active power P and reactive power Q  associated with a periodic set of 3-phase voltages and currents which may contain harmonics. P and Q are calculated by evaluating the fundamental values (positive-sequence) of the input voltages and currents with a running window over one cycle of the specified frequency (port Freq).
      |  Input port "Sin_Cos" (a two-dimension signal) provides the reference frame required for the computation.
      |
      | input 1: must give the frequency of the fundamental (Hz)
      | Input 2: must contain a  [sin(wt)  cos(wt)] two dimension signal , where w is the rotation speed (rad/s) of the reference frame used for the computation..
      | input 3: Vectorized 3-phase  instantaneous voltage (Vabc)
      | input 4: Vectorized 3-phase instantaneous current (Iabc)
      |
      | Output 1: Vector [Mag_V Mag_I] of the fundamental values (Magnitude) of the voltage & current (peak values of the positive-sequence)
      | Output 2: 3-phase PQ measurement vector [P(W) Q (var)] evaluated at the specified frequency. Current flowing into an RL circuit will produce  positive active and reactive powers.
      |
      | For the first cycle of simulation, the outputs are held constant using the values specified by the parameters "Initial input".
      | he value of the parameter "Minimum frequency" is used to determine the buffer size of the "Variable Transport Delay" block found inside this subsystem.
      mask init:
      | power_initmask();
      settings: OpenFcn=power_openblockproxy();
  Divide : Product  Inputs=*/
  Filter : Subsystem  mask{Freq=Freq_filter, Zeta=Zeta_filter, Ts=Ts}
      mask prompts: Freq "Cut-off frequency (Hz):"; Zeta "Damping factor Zeta:"; Ts "Sample time"
  Gain : Gain  Gain=1.4
  Less Than : RelationalOperator  Operator=>  OutDataTypeStr=boolean  RndMeth=Simplest
  Less Than1 : RelationalOperator  Operator=>  OutDataTypeStr=boolean  RndMeth=Simplest
  Logical Operator : Logic  AllPortsSameDT=off  OutDataTypeStr=boolean
  Math Function1 : Math  Operator=square  SaturateOnIntegerOverflow=on
  Max : MinMax  Inputs=2
  Memory : Memory  InitialCondition=1
  Second-Order Filter1 : powerlib_meascontrol/Filters/Second-Order Filter  FilterType=Lowpass  Fo=50  Zeta=0.707  Ts=Ts  Initialize=off  Vac_Init="[0,  0,  60]"  Vdc_Init=0  PlotResponse=off  FreqRange=[0, 500, 1]
      settings: SourceProductBaseCode=PS
  Selector1 : Selector  InputPortWidth=2  IndexOptions=Index vector (dialog)  Indices=1  OutputSizes=1
  Selector2 : Selector  InputPortWidth=2  IndexOptions=Index vector (dialog)  Indices=1  OutputSizes=1
  Selector3 : Selector  InputPortWidth=2  IndexOptions=Index vector (dialog)  Indices=2  OutputSizes=1
  "Sinusoidal Measurement (PLL, Three-Phase)" : eeSinusoidalMeasurement/Sinusoidal Measurement (PLL, Three-Phase)  Kp_LF=200*0.1  Ki_LF=2000*0.1  F0=freq  Theta0=0  Ts=-1
      settings: SourceProductBaseCode=PS
  Sum : Sum  Inputs=|-+
  Sum1 : Sum  Inputs=|++
  Switch1 : Switch  Criteria=u2 > Threshold
  Switch2 : Switch  Criteria=u2 > Threshold
  Terminator : Terminator
  V->pu : Gain  Gain=1/(Vnom/sqrt(3)*sqrt(2))  SaturateOnIntegerOverflow=on  OutDataTypeStr=Inherit: Same as input  ParamDataTypeStr=Inherit: Same as input
  W->pu : Gain  Gain=-1/Pnom  SaturateOnIntegerOverflow=on  OutDataTypeStr=Inherit: Same as input  ParamDataTypeStr=Inherit: Same as input
  pu->A : Gain  Gain=Pnom/sqrt(3)/Vnom*sqrt(2)  SaturateOnIntegerOverflow=on  OutDataTypeStr=Inherit: Same as input  ParamDataTypeStr=Inherit: Same as input
  pu->V : Gain  Gain=Vnom/sqrt(3)*sqrt(2)  SaturateOnIntegerOverflow=on  OutDataTypeStr=Inherit: Same as input  ParamDataTypeStr=Inherit: Same as input
  "var->pu " : Gain  Gain=-1/Pnom  SaturateOnIntegerOverflow=on  OutDataTypeStr=Inherit: Same as input  ParamDataTypeStr=Inherit: Same as input
  "IL " : Outport  VectorParamsAs1DForOutWhenUnconnected=on
  Theta_PLL : Outport  Port=2  VectorParamsAs1DForOutWhenUnconnected=on
  Pmeas : Outport  Port=3  VectorParamsAs1DForOutWhenUnconnected=on
  Qmeas : Outport  Port=4  VectorParamsAs1DForOutWhenUnconnected=on
  Vmag : Outport  Port=5  VectorParamsAs1DForOutWhenUnconnected=on
  Vdc_meas : Outport  Port=6  VectorParamsAs1DForOutWhenUnconnected=on
  Qref_pu : Outport  Port=7  VectorParamsAs1DForOutWhenUnconnected=on
  Vnormal : Outport  Port=8  VectorParamsAs1DForOutWhenUnconnected=on
  wires:
  [IL] -> "IL "/1
  Filter/3("IL ") -> [IL]
  IL/1 -> Filter/3(IL)
  Sum1/1 -> W->pu/1
  C_var_filter/Q/1 -> Sum1/2
  Selector1/1 -> Sum1/1
  Math Function1/1 -> C_var_filter/1, C_var_filter/Q/1
  Sum/1 -> "var->pu "/1  "Q meas"
  C_var_filter/1 -> Sum/1
  Selector3/1 -> Sum/2  "Q grid"
  Divide/1 -> Math Function1/1
  Constant1/1 -> Divide/2
  [V_volt] -> Divide/1
  Iabc_gc/1 -> Filter/2(Iabc_grid_conv)
  Filter/5("Qref ") -> [Qref]
  Filter/4("Vdc ") -> [Vdc_meas]
  Filter/2("Iabc_grid_conv ") -> [Iabc_gc]
  Filter/1("Vabc_grid ") -> [Vabc_grid]
  Qref/1 -> Filter/5(Qref)
  Vdc/1 -> Filter/4(Vdc)
  Vabc_grid/1 -> Filter/1(Vabc_grid)
  Discrete 3-phase PLL-Driven Positive-Sequence Active & Reactive Power/2(P_Q) -> [PQ]
  [Iabc_gc] -> pu->A/1
  [Qref] -> Qref_pu/1
  [Vdc_meas] -> Vdc_meas/1
  [PQ] -> Selector1/1
  pu->A/1 -> Discrete 3-phase PLL-Driven Positive-Sequence Active & Reactive Power/4(Iabc)
  [Vmeas] -> Vmag/1
  [Pmeas] -> Pmeas/1
  [Theta] -> Theta_PLL/1
  [Vabc_grid] -> "Sinusoidal Measurement (PLL, Three-Phase)"/1
  [Theta] -> Discrete 3-phase PLL-Driven Positive-Sequence Active & Reactive Power/2(w)
  "Sinusoidal Measurement (PLL, Three-Phase)"/2 -> [Theta]
  W->pu/1 -> [Pmeas]
  pu->V/1 -> Discrete 3-phase PLL-Driven Positive-Sequence Active & Reactive Power/3(Vabc)
  "Sinusoidal Measurement (PLL, Three-Phase)"/1 -> [Freq]
  Discrete 3-phase PLL-Driven Positive-Sequence Active & Reactive Power/1(Mag_V_I) -> Selector2/1
  [V_volt] -> V->pu/1
  V->pu/1 -> [Vmeas]
  [PQ] -> Selector3/1
  "var->pu "/1 -> [Qmeas]  "Q meas pu"
  [Qmeas] -> Qmeas/1
  "Sinusoidal Measurement (PLL, Three-Phase)"/3 -> Terminator/1
  Selector2/1 -> [V_volt]  "V volt"
  [Vabc_grid] -> pu->V/1
  [Vnormal] -> Vnormal/1
  [Freq] -> Discrete 3-phase PLL-Driven Positive-Sequence Active & Reactive Power/1(Freq)
  [V_volt] -> Second-Order Filter1/1
  Constant2/1 -> Less Than1/2  "20 Hz"
  [Freq] -> Less Than1/1  "Freq"
  Memory/1 -> Max/2
  Gain/1 -> Less Than/1
  Second-Order Filter1/1 -> Less Than/2
  Constant/1 -> Gain/1
  Max/1 -> [Vnormal], Memory/1
  Logical Operator/1 -> Max/1
  Constant3/1 -> Switch2/1
  Digital Clock1/1 -> Compare To Constant3/1
  Compare To Constant3/1 -> Switch2/2
  Less Than/1 -> Switch2/3
  Switch2/1 -> Logical Operator/1  "test1"
  Digital Clock2/1 -> Compare To Constant1/1
  Constant4/1 -> Switch1/1
  Less Than1/1 -> Switch1/3  "Comparator freq"
  Switch1/1 -> Logical Operator/2  "test2"
  Compare To Constant1/1 -> Switch1/2

== system Farm_FaultBottomBar/SM_WT1/Wind Type IV Detailed v2.1 - 3/Control/PI_P ==
  u : Inport
  Enable : EnablePort
  Discrete PID Controller2 : simulink/Continuous/PID Controller  Controller=PI  Form=Parallel  TimeDomain=Discrete-time  SampleTime=-1  IntegratorMethod=Forward Euler  FilterMethod=Forward Euler  ControllerParametersSource=internal  P=5  I=30  D=2  UseFilter=on  N=100  TunerSelectOption=Transfer Function Based (PID Tuner App)  InitialConditionSource=internal  InitialConditionForIntegrator=0  InitialConditionForFilter=0  DifferentiatorICPrevScaledInput=0  ExternalReset=none  TrackingMode=off  Kt=1  LimitOutput=on  UpperSaturationLimit=0.8  LowerSaturationLimit=-0.8  LinearizeAsGain=off  AntiWindupMode=none  Kb=1  POutMin=[]  POutMax=[]  IOutMin=[]  IOutMax=[]  DOutMin=[]  DOutMax=[]  NOutMin=[]  NOutMax=[]  SumOutMin=[]  SumOutMax=[]  SaturationOutMin=[]  SaturationOutMax=[]  PParamMin=[]  PParamMax=[]  IParamMin=[]  IParamMax=[]  DParamMin=[]  DParamMax=[]  NParamMin=[]  NParamMax=[]  KbParamMin=[]  KbParamMax=[]  KtParamMin=[]  KtParamMax=[]  KbOutMin=[]  KbOutMax=[]  KtOutMin=[]  KtOutMax=[]  IntegratorOutMin=[]  IntegratorOutMax=[]  FilterOutMin=[]  FilterOutMax=[]  SumI1OutMin=[]  SumI1OutMax=[]  SumI2OutMin=[]  SumI2OutMax=[]  SumI3OutMin=[]  SumI3OutMax=[]  SumI4OutMin=[]  SumI4OutMax=[]  SumDOutMin=[]  SumDOutMax=[]  DifferentiatorOutMin=[]  DifferentiatorOutMax=[]  FilterDiffOutCoefMin=[]  FilterDiffOutCoefMax=[]  ReciprocalOutMin=[]  ReciprocalOutMax=[]  SumDenOutMin=[]  SumDenOutMax=[]  SumNumOutMin=[]  SumNumOutMax=[]  DivideOutMin=[]  DivideOutMax=[]  IntegratorContinuousStateAttributes=''  IntegratorStateMustResolveToSignalObject=off  IntegratorRTWStateStorageClass=Auto  FilterContinuousStateAttributes=''  FilterStateMustResolveToSignalObject=off  FilterRTWStateStorageClass=Auto  ParallelPVariant=InternalParameters  IdealPVariant=Disabled  IVariant=InternalParameters  DVariant=Disabled  IntegratorVariant=Discrete  SatVariant=Enabled  AWVariant=Passthrough  PCopyVariant=Disabled  TRVariant=Disabled  FdbkBlocksVariant=Forward  IdealPFdbkVariant=Disabled  SatFdbkVariant=Disabled  DerivativeFilterVariant=Disabled  NVariant=Disabled  NCopyVariant=Disabled_SignalSpec  FilterICVariant=Disabled  IntegratorICVariant=InternalICs  ExternalResetVariant=Disabled  TRSumVariant=Passthrough  SumFdbkVariant=Disabled  SumVariant=Sum_PI
  PI_out : Outport  VectorParamsAs1DForOutWhenUnconnected=on
  wires:
  Discrete PID Controller2/1 -> PI_out/1  "d PI_out"
  u/1 -> Discrete PID Controller2/1

== system Farm_FaultBottomBar/SM_WT1/Wind Type IV Detailed v2.1 - 3/Control/PI_Q ==
  Qerr : Inport
  Enable : EnablePort
  Discrete PID Controller1 : simulink/Continuous/PID Controller  Controller=PI  Form=Parallel  TimeDomain=Discrete-time  SampleTime=-1  IntegratorMethod=Forward Euler  FilterMethod=Forward Euler  ControllerParametersSource=internal  P=0.5  I=8  D=2  UseFilter=on  N=100  TunerSelectOption=Transfer Function Based (PID Tuner App)  InitialConditionSource=internal  InitialConditionForIntegrator=0  InitialConditionForFilter=0  DifferentiatorICPrevScaledInput=0  ExternalReset=none  TrackingMode=off  Kt=1  LimitOutput=off  UpperSaturationLimit=inf  LowerSaturationLimit=-inf  LinearizeAsGain=off  AntiWindupMode=none  Kb=1  POutMin=[]  POutMax=[]  IOutMin=[]  IOutMax=[]  DOutMin=[]  DOutMax=[]  NOutMin=[]  NOutMax=[]  SumOutMin=[]  SumOutMax=[]  SaturationOutMin=[]  SaturationOutMax=[]  PParamMin=[]  PParamMax=[]  IParamMin=[]  IParamMax=[]  DParamMin=[]  DParamMax=[]  NParamMin=[]  NParamMax=[]  KbParamMin=[]  KbParamMax=[]  KtParamMin=[]  KtParamMax=[]  KbOutMin=[]  KbOutMax=[]  KtOutMin=[]  KtOutMax=[]  IntegratorOutMin=[]  IntegratorOutMax=[]  FilterOutMin=[]  FilterOutMax=[]  SumI1OutMin=[]  SumI1OutMax=[]  SumI2OutMin=[]  SumI2OutMax=[]  SumI3OutMin=[]  SumI3OutMax=[]  SumI4OutMin=[]  SumI4OutMax=[]  SumDOutMin=[]  SumDOutMax=[]  DifferentiatorOutMin=[]  DifferentiatorOutMax=[]  FilterDiffOutCoefMin=[]  FilterDiffOutCoefMax=[]  ReciprocalOutMin=[]  ReciprocalOutMax=[]  SumDenOutMin=[]  SumDenOutMax=[]  SumNumOutMin=[]  SumNumOutMax=[]  DivideOutMin=[]  DivideOutMax=[]  IntegratorContinuousStateAttributes=''  IntegratorStateMustResolveToSignalObject=off  IntegratorRTWStateStorageClass=Auto  FilterContinuousStateAttributes=''  FilterStateMustResolveToSignalObject=off  FilterRTWStateStorageClass=Auto  ParallelPVariant=InternalParameters  IdealPVariant=Disabled  IVariant=InternalParameters  DVariant=Disabled  IntegratorVariant=Discrete  SatVariant=Disabled  AWVariant=Passthrough  PCopyVariant=Disabled  TRVariant=Disabled  FdbkBlocksVariant=Forward  IdealPFdbkVariant=Disabled  SatFdbkVariant=Disabled  DerivativeFilterVariant=Disabled  NVariant=Disabled  NCopyVariant=Disabled_SignalSpec  FilterICVariant=Disabled  IntegratorICVariant=InternalICs  ExternalResetVariant=Disabled  TRSumVariant=Passthrough  SumFdbkVariant=Disabled  SumVariant=Sum_PI
  PI_out : Outport  VectorParamsAs1DForOutWhenUnconnected=on
  wires:
  Discrete PID Controller1/1 -> PI_out/1  "q PI_out"
  Qerr/1 -> Discrete PID Controller1/1

== system Farm_FaultBottomBar/SM_WT1/Wind Type IV Detailed v2.1 - 3/Control/Pulse Generator1 ==
  Duty_Cycle : Inport
  Add : Sum  Inputs=-+
  Constant3 : Constant
  Constant4 : Constant  Value=0
  Digital Clock : DigitalClock  SampleTime=Ts
  Divide2 : Product  Inputs=**
  Divide3 : Product  Inputs=**
  Math Function : Math  Operator=mod  SaturateOnIntegerOverflow=on
  Nb_of_samples_by_cycle : Constant  Value=1/Freq_sawtooth/Ts
  Relational Operator1 : RelationalOperator  Operator=>  OutDataTypeStr=boolean  RndMeth=Nearest
  Rounding Function1 : Rounding  Operator=round
  Switch : Switch  Threshold=0.5
  Ts : Constant  Value=Ts
  Pulse : Outport  VectorParamsAs1DForOutWhenUnconnected=on
  wires:
  Switch/1 -> Pulse/1
  Add/1 -> Divide2/2
  Digital Clock/1 -> Math Function/1
  Ts/1 -> Add/1, Divide3/1
  Rounding Function1/1 -> Divide3/2  "Nb_of_samples_by_cycle"
  Duty_Cycle/1 -> Divide2/1
  Divide3/1 -> Math Function/2, Add/2  "Period_of_cycle"
  Divide2/1 -> Relational Operator1/1
  Nb_of_samples_by_cycle/1 -> Rounding Function1/1
  Relational Operator1/1 -> Switch/2
  Constant3/1 -> Switch/1
  Constant4/1 -> Switch/3
  Math Function/1 -> Relational Operator1/2

== system Farm_FaultBottomBar/SM_WT1/Wind Type IV Detailed v2.1 - 33/AC fault ride though characteristic/Triggered Subsystem ==
  In1 : Inport
  Trigger : TriggerPort  VariantControl=Variant
  Time_trigger_FRT : Outport  VectorParamsAs1DForOutWhenUnconnected=on
  wires:
  In1/1 -> Time_trigger_FRT/1

== system Farm_FaultBottomBar/SM_WT1/Wind Type IV Detailed v2.1 - 33/Control/2 sample av. ==
  in : Inport
  Delay : Delay  DelayLength=1  InitialCondition=Init_value  SampleTime=Ts
  Delay1 : Delay  DelayLength=1  InitialCondition=Init_value  SampleTime=Ts
  Gain : Gain  Gain=0.5
  Sum1 : Sum  Inputs=|++
  out : Outport
  wires:
  Gain/1 -> out/1
  in/1 -> Delay/1
  Delay1/1 -> Sum1/2
  Sum1/1 -> Gain/1
  Delay/1 -> Delay1/1, Sum1/1
